simulink model "Simulations_Ex_2_3_4_5"  (R2016b)
settings: Solver=VariableStepAuto  StartTime=0.0  StopTime=25  RelTol=1e-3
libraries: powerlib_meascontrol x5
settings Model: Creator=CBalla  LastModifiedBy=CBalla

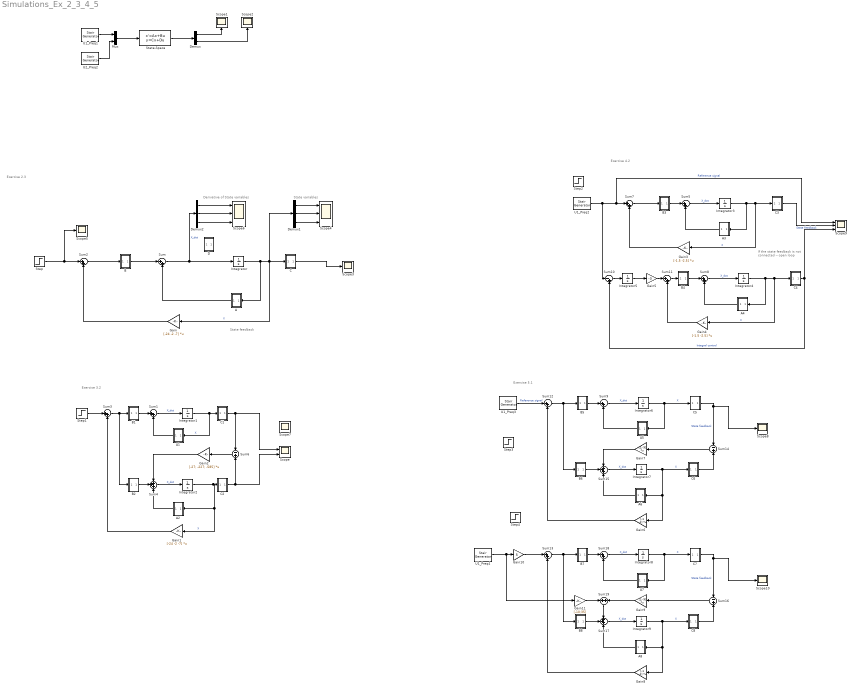
== system Simulations_Ex_2_3_4_5 ==
  note: If the state feedback is not
      | connected -- open loop
  note: Exercise 2.3
  note: State feedback
  note: Derivative of State variables
  note: State variables
  note: Exercise 3.2
  note: Exercise 4.2
  note: Exercise 5.1
  A : Subsystem
      mask Display:
      | %color('cyan')
      | color('magenta')
      | disp('{\bf\fontsize{14}A}', 'texmode','on');
      | %disp('B')
  A1 : Subsystem
      mask Display:
      | %color('cyan')
      | color('magenta')
      | disp('{\bf\fontsize{14}A}', 'texmode','on');
      | %disp('B')
  A2 : Subsystem
      mask Display:
      | %color('cyan')
      | color('magenta')
      | disp('{\bf\fontsize{14}A}', 'texmode','on');
      | %disp('B')
  A3 : Subsystem
      mask Display:
      | %color('cyan')
      | color('magenta')
      | disp('{\bf\fontsize{14}A}', 'texmode','on');
      | %disp('B')
  A4 : Subsystem
      mask Display:
      | %color('cyan')
      | color('magenta')
      | disp('{\bf\fontsize{14}A}', 'texmode','on');
      | %disp('B')
  A5 : Subsystem
      mask Display:
      | %color('cyan')
      | color('magenta')
      | disp('{\bf\fontsize{14}A}', 'texmode','on');
      | %disp('B')
  A6 : Subsystem
      mask Display:
      | %color('cyan')
      | color('magenta')
      | disp('{\bf\fontsize{14}A}', 'texmode','on');
      | %disp('B')
  A7 : Subsystem
      mask Display:
      | %color('cyan')
      | color('magenta')
      | disp('{\bf\fontsize{14}A}', 'texmode','on');
      | %disp('B')
  A8 : Subsystem
      mask Display:
      | %color('cyan')
      | color('magenta')
      | disp('{\bf\fontsize{14}A}', 'texmode','on');
      | %disp('B')
  B : Subsystem
      mask Display:
      | %color('cyan')
      | color('magenta')
      | disp('{\bf\fontsize{14}B}', 'texmode','on');
      | %disp('B')
  B1 : Subsystem
      mask Display:
      | %color('cyan')
      | color('magenta')
      | disp('{\bf\fontsize{14}B}', 'texmode','on');
      | %disp('B')
  B2 : Subsystem
      mask Display:
      | %color('cyan')
      | color('magenta')
      | disp('{\bf\fontsize{14}B}', 'texmode','on');
      | %disp('B')
  B3 : Subsystem
      mask Display:
      | %color('cyan')
      | color('magenta')
      | disp('{\bf\fontsize{14}B}', 'texmode','on');
      | %disp('B')
  B4 : Subsystem
      mask Display:
      | %color('cyan')
      | color('magenta')
      | disp('{\bf\fontsize{14}B}', 'texmode','on');
      | %disp('B')
  B5 : Subsystem
      mask Display:
      | %color('cyan')
      | color('magenta')
      | disp('{\bf\fontsize{14}B}', 'texmode','on');
      | %disp('B')
  B6 : Subsystem
      mask Display:
      | %color('cyan')
      | color('magenta')
      | disp('{\bf\fontsize{14}B}', 'texmode','on');
      | %disp('B')
  B7 : Subsystem
      mask Display:
      | %color('cyan')
      | color('magenta')
      | disp('{\bf\fontsize{14}B}', 'texmode','on');
      | %disp('B')
  B8 : Subsystem
      mask Display:
      | %color('cyan')
      | color('magenta')
      | disp('{\bf\fontsize{14}B}', 'texmode','on');
      | %disp('B')
  C : Subsystem
      mask Display:
      | %color('cyan')
      | color('magenta')
      | disp('{\bf\fontsize{14}C}', 'texmode','on');
      | %disp('B')
  C1 : Subsystem
      mask Display:
      | %color('cyan')
      | color('magenta')
      | disp('{\bf\fontsize{14}C}', 'texmode','on');
      | %disp('B')
  C2 : Subsystem
      mask Display:
      | %color('cyan')
      | color('magenta')
      | disp('{\bf\fontsize{14}C}', 'texmode','on');
      | %disp('B')
  C3 : Subsystem
      mask Display:
      | %color('cyan')
      | color('magenta')
      | disp('{\bf\fontsize{14}C}', 'texmode','on');
      | %disp('B')
  C4 : Subsystem
      mask Display:
      | %color('cyan')
      | color('magenta')
      | disp('{\bf\fontsize{14}C}', 'texmode','on');
      | %disp('B')
  C5 : Subsystem
      mask Display:
      | %color('cyan')
      | color('magenta')
      | disp('{\bf\fontsize{14}C}', 'texmode','on');
      | %disp('B')
  C6 : Subsystem
      mask Display:
      | %color('cyan')
      | color('magenta')
      | disp('{\bf\fontsize{14}C}', 'texmode','on');
      | %disp('B')
  C7 : Subsystem
      mask Display:
      | %color('cyan')
      | color('magenta')
      | disp('{\bf\fontsize{14}C}', 'texmode','on');
      | %disp('B')
  C8 : Subsystem
      mask Display:
      | %color('cyan')
      | color('magenta')
      | disp('{\bf\fontsize{14}C}', 'texmode','on');
      | %disp('B')
  D : Subsystem
      mask Display:
      | %color('cyan')
      | color('magenta')
      | disp('{\bf\fontsize{14}D}', 'texmode','on');
      | %disp('B')
  Demux : Demux  Outputs=2
  Demux1 : Demux  Outputs=3
  Demux2 : Demux  Outputs=3
  Gain : Gain  Gain=[-24 -2 -7]  Multiplication=Matrix(K*u)
  Gain1 : Gain  Gain=[-24 -2 -7]  Multiplication=Matrix(K*u)
  Gain10 : Gain  Gain=5
  Gain11 : Gain  Gain=[-10;35]
  Gain2 : Gain  Gain=[-27; -227; -585]  Multiplication=Matrix(K*u)
  Gain3 : Gain  Gain=[-1.5 -2.5]  Multiplication=Matrix(K*u)
  Gain4 : Gain  Gain=[-1.5 -2.5]  Multiplication=Matrix(K*u)
  Gain5 : Gain  Gain=-3
  Gain6 : Gain  Gain=[-1 -1]  Multiplication=Matrix(K*u)
  Gain7 : Gain  Gain=[2;-9]  Multiplication=Matrix(K*u)
  Gain8 : Gain  Gain=[-1 -1]  Multiplication=Matrix(K*u)
  Gain9 : Gain  Gain=[2;-9]  Multiplication=Matrix(K*u)
  Integrator{,2..9} (9 alike) : Integrator
  Integrator1 : Integrator  InitialCondition=-1
  Mux : Mux  Inputs=2
  Scope : Scope  NumInputPorts=2
  Scope{1..3,5,7..8,10} (7 alike) : Scope
  Scope4 : Scope  NumInputPorts=3
  Scope6 : Scope  NumInputPorts=3
  Scope9 : Scope  NumInputPorts=3
  State-Space : StateSpace  A=[-5.2159 -79.1175 -0.7209 -0.7209; 1 0 0 0; 0 0 -1.4430 -0.7209; 0 0 1 0]  B=|  C=|  D=[0.9645 0; 0 0]  X0=0
      B=|
      | [1 0;
      | 0 0;
      | 0 1; 0 0]
      C=|
      | [-1.3307 2.8087 -0.69530805 -0.69530805;
      | 0 0 0.7209 0.7209]
  Step{,1..4} (5 alike) : Step  Time=3  SampleTime=0
  Sum{,1..3,5,7..9,11..13,18} (12 alike) : Sum  Inputs=|++
  Sum10 : Sum  Inputs=|-+
  Sum14 : Sum  Inputs=-+
  Sum15 : Sum  Inputs=+++
  Sum16 : Sum  Inputs=-+
  Sum17 : Sum  Inputs=+++
  Sum19 : Sum
  Sum4 : Sum  Inputs=+++
  Sum6 : Sum  Inputs=-+
  U1_Preq1 : powerlib_meascontrol/Pulse & Signal Generators/Stair Generator  t=[4, 7, 12, 18,25]  e=[10000, 11500, 2000, 15000,2000]  Ts=0
  U1_Preq2 : powerlib_meascontrol/Pulse & Signal Generators/Stair Generator  t=[1, 4, 10, 15,20]  e=[1, 0, 2, -1,0]  Ts=0
  U1_Preq3 : powerlib_meascontrol/Pulse & Signal Generators/Stair Generator  t=[1, 4, 10, 15,20]  e=[1, 0, 2, -1,0]  Ts=0
  U1_Preq4 : powerlib_meascontrol/Pulse & Signal Generators/Stair Generator  t=[1, 4, 10, 15,20]  e=[1, 0, 2, -1,0]  Ts=0
  U2_Preq2 : powerlib_meascontrol/Pulse & Signal Generators/Stair Generator  t=[10, 18,25]  e=[10000, 15000,2000]  Ts=0
  wires:
  U1_Preq1/1 -> Mux/1
  U2_Preq2/1 -> Mux/2
  Mux/1 -> State-Space/1
  State-Space/1 -> Demux/1
  Demux/1 -> Scope1/1
  Demux/2 -> Scope2/1
  B/1(Out1) -> Sum/1
  A/1(Out1) -> Sum/2
  Demux2/1 -> Scope6/1
  Demux2/2 -> Scope6/2
  Demux2/3 -> Scope6/3
  Sum2/1 -> B/1(In1)
  Integrator/1 -> Demux1/1, Gain/1, C/1(In1), A/1(In1)  "X"
  Gain/1 -> Sum2/2
  Sum/1 -> Demux2/1, Integrator/1  "X_dot"
  C/1(Out1) -> Scope3/1
  Step/1 -> Scope5/1, Sum2/1
  Demux1/2 -> Scope4/2
  Demux1/3 -> Scope4/3
  Demux1/1 -> Scope4/1
  B1/1(Out1) -> Sum1/1
  A1/1(Out1) -> Sum1/2
  Sum3/1 -> B2/1(In1), B1/1(In1)
  Integrator1/1 -> C1/1(In1), A1/1(In1)  "X"
  Sum1/1 -> Integrator1/1  "X_dot"
  C1/1(Out1) -> Sum6/1, Scope/1
  Step1/1 -> Sum3/1
  Integrator2/1 -> Gain1/1, A2/1(In1), C2/1(In1)  "X"
  Sum4/1 -> Integrator2/1  "X_dot"
  C2/1(Out1) -> Scope/2, Sum6/2
  Gain1/1 -> Sum3/2
  Sum6/1 -> Gain2/1
  A2/1(Out1) -> Sum4/3
  B2/1(Out1) -> Sum4/2
  Gain2/1 -> Sum4/1
  B3/1(Out1) -> Sum5/1
  A3/1(Out1) -> Sum5/2
  Sum7/1 -> B3/1(In1)
  Integrator3/1 -> Gain3/1, C3/1(In1), A3/1(In1)  "X"
  Sum5/1 -> Integrator3/1  "X_dot"
  U1_Preq2/1 -> Sum10/1, Scope9/1, Sum7/1  "Reference signal"
  C3/1(Out1) -> Scope9/2  "State feedback"
  B4/1(Out1) -> Sum8/1
  A4/1(Out1) -> Sum8/2
  Sum10/1 -> Integrator5/1
  Integrator4/1 -> Gain4/1, C4/1(In1), A4/1(In1)  "X"
  Sum8/1 -> Integrator4/1  "X_dot"
  Integrator5/1 -> Gain5/1
  Gain5/1 -> Sum11/1
  Sum11/1 -> B4/1(In1)
  Gain4/1 -> Sum11/2
  C4/1(Out1) -> Scope9/3, Sum10/2  "Integral control"
  Gain3/1 -> Sum7/2
  B5/1(Out1) -> Sum9/1
  A5/1(Out1) -> Sum9/2
  Integrator6/1 -> C5/1(In1), A5/1(In1)  "X"
  Sum9/1 -> Integrator6/1  "X_dot"
  B6/1(Out1) -> Sum15/2
  Sum12/1 -> B6/1(In1), B5/1(In1)
  Integrator7/1 -> C6/1(In1), Gain6/1, A6/1(In1)  "X"
  Sum15/1 -> Integrator7/1  "X_dot"
  C5/1(Out1) -> Scope8/1, Sum14/1  "State feedback"
  C6/1(Out1) -> Sum14/2
  Sum14/1 -> Gain7/1
  A6/1(Out1) -> Sum15/3
  Gain7/1 -> Sum15/1
  Gain6/1 -> Sum12/2
  B7/1(Out1) -> Sum18/1
  A7/1(Out1) -> Sum18/2
  Integrator8/1 -> C7/1(In1), A7/1(In1)  "X"
  Sum18/1 -> Integrator8/1  "X_dot"
  B8/1(Out1) -> Sum17/2
  Sum13/1 -> B8/1(In1), B7/1(In1)
  Integrator9/1 -> C8/1(In1), Gain8/1, A8/1(In1)  "X"
  Sum17/1 -> Integrator9/1  "X_dot"
  C7/1(Out1) -> Scope10/1, Sum16/1  "State feedback"
  C8/1(Out1) -> Sum16/2
  Sum16/1 -> Gain9/1
  A8/1(Out1) -> Sum17/3
  Gain8/1 -> Sum13/2
  U1_Preq3/1 -> Sum12/1  "Reference signal"
  U1_Preq4/1 -> Gain11/1, Gain10/1
  Gain10/1 -> Sum13/1
  Sum19/1 -> Sum17/1
  Gain9/1 -> Sum19/2
  Gain11/1 -> Sum19/1

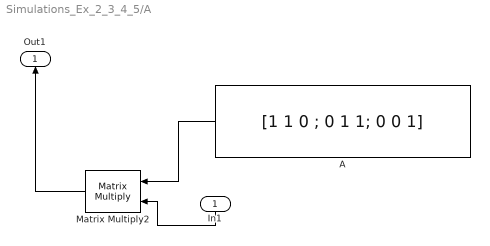
== system Simulations_Ex_2_3_4_5/A ==
  In1 : Inport
  A : Constant  Value=[1 1 0 ; 0 1 1; 0 0 1]  VectorParams1D=off
  Matrix Multiply2 : Product  Multiplication=Matrix(*)
  Out1 : Outport
  wires:
  Matrix Multiply2/1 -> Out1/1
  A/1 -> Matrix Multiply2/1
  In1/1 -> Matrix Multiply2/2

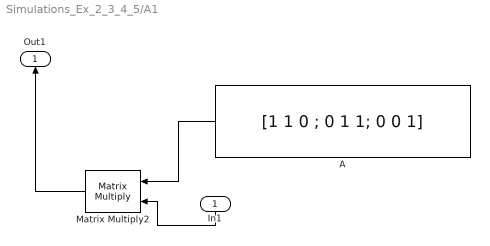
== system Simulations_Ex_2_3_4_5/A1 ==
  In1 : Inport
  A : Constant  Value=[1 1 0 ; 0 1 1; 0 0 1]  VectorParams1D=off
  Matrix Multiply2 : Product  Multiplication=Matrix(*)
  Out1 : Outport
  wires:
  Matrix Multiply2/1 -> Out1/1
  A/1 -> Matrix Multiply2/1
  In1/1 -> Matrix Multiply2/2

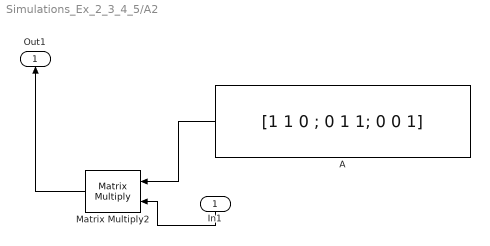
== system Simulations_Ex_2_3_4_5/A2 ==
  In1 : Inport
  A : Constant  Value=[1 1 0 ; 0 1 1; 0 0 1]  VectorParams1D=off
  Matrix Multiply2 : Product  Multiplication=Matrix(*)
  Out1 : Outport
  wires:
  Matrix Multiply2/1 -> Out1/1
  A/1 -> Matrix Multiply2/1
  In1/1 -> Matrix Multiply2/2

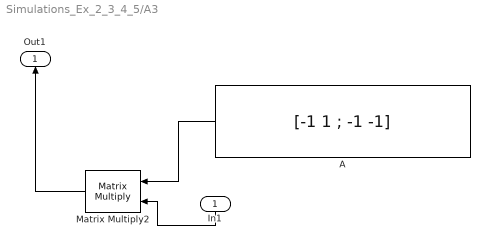
== system Simulations_Ex_2_3_4_5/A3 ==
  In1 : Inport
  A : Constant  Value=[-1 1 ; -1 -1]  VectorParams1D=off
  Matrix Multiply2 : Product  Multiplication=Matrix(*)
  Out1 : Outport
  wires:
  Matrix Multiply2/1 -> Out1/1
  A/1 -> Matrix Multiply2/1
  In1/1 -> Matrix Multiply2/2

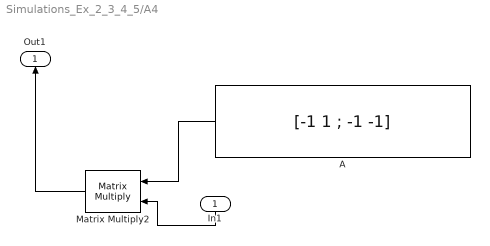
== system Simulations_Ex_2_3_4_5/A4 ==
  In1 : Inport
  A : Constant  Value=[-1 1 ; -1 -1]  VectorParams1D=off
  Matrix Multiply2 : Product  Multiplication=Matrix(*)
  Out1 : Outport
  wires:
  Matrix Multiply2/1 -> Out1/1
  A/1 -> Matrix Multiply2/1
  In1/1 -> Matrix Multiply2/2

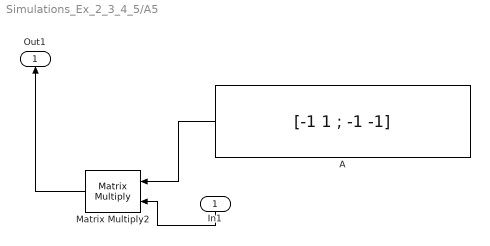
== system Simulations_Ex_2_3_4_5/A5 ==
  In1 : Inport
  A : Constant  Value=[-1 1 ; -1 -1]  VectorParams1D=off
  Matrix Multiply2 : Product  Multiplication=Matrix(*)
  Out1 : Outport
  wires:
  Matrix Multiply2/1 -> Out1/1
  A/1 -> Matrix Multiply2/1
  In1/1 -> Matrix Multiply2/2

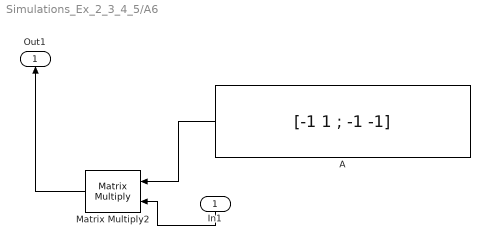
== system Simulations_Ex_2_3_4_5/A6 ==
  In1 : Inport
  A : Constant  Value=[-1 1 ; -1 -1]  VectorParams1D=off
  Matrix Multiply2 : Product  Multiplication=Matrix(*)
  Out1 : Outport
  wires:
  Matrix Multiply2/1 -> Out1/1
  A/1 -> Matrix Multiply2/1
  In1/1 -> Matrix Multiply2/2

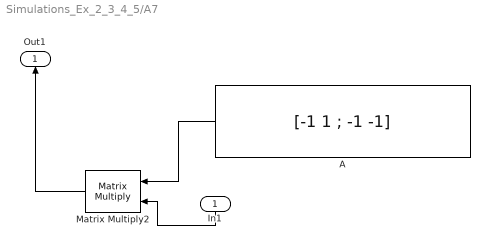
== system Simulations_Ex_2_3_4_5/A7 ==
  In1 : Inport
  A : Constant  Value=[-1 1 ; -1 -1]  VectorParams1D=off
  Matrix Multiply2 : Product  Multiplication=Matrix(*)
  Out1 : Outport
  wires:
  Matrix Multiply2/1 -> Out1/1
  A/1 -> Matrix Multiply2/1
  In1/1 -> Matrix Multiply2/2

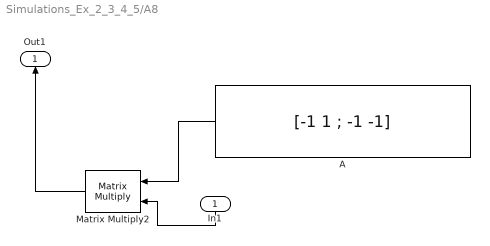
== system Simulations_Ex_2_3_4_5/A8 ==
  In1 : Inport
  A : Constant  Value=[-1 1 ; -1 -1]  VectorParams1D=off
  Matrix Multiply2 : Product  Multiplication=Matrix(*)
  Out1 : Outport
  wires:
  Matrix Multiply2/1 -> Out1/1
  A/1 -> Matrix Multiply2/1
  In1/1 -> Matrix Multiply2/2

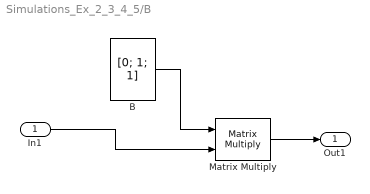
== system Simulations_Ex_2_3_4_5/B ==
  In1 : Inport
  B : Constant  Value=|  VectorParams1D=off
      | [0;
      | 1;
      | 1]
  Matrix Multiply : Product  Multiplication=Matrix(*)
  Out1 : Outport
  wires:
  Matrix Multiply/1 -> Out1/1
  B/1 -> Matrix Multiply/1
  In1/1 -> Matrix Multiply/2

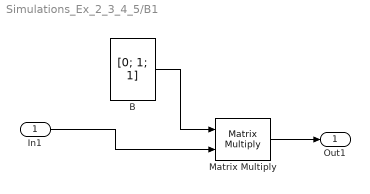
== system Simulations_Ex_2_3_4_5/B1 ==
  In1 : Inport
  B : Constant  Value=|  VectorParams1D=off
      | [0;
      | 1;
      | 1]
  Matrix Multiply : Product  Multiplication=Matrix(*)
  Out1 : Outport
  wires:
  Matrix Multiply/1 -> Out1/1
  B/1 -> Matrix Multiply/1
  In1/1 -> Matrix Multiply/2

== system Simulations_Ex_2_3_4_5/B2 ==
  In1 : Inport
  B : Constant  Value=|  VectorParams1D=off
      | [0;
      | 1;
      | 1]
  Matrix Multiply : Product  Multiplication=Matrix(*)
  Out1 : Outport
  wires:
  Matrix Multiply/1 -> Out1/1
  B/1 -> Matrix Multiply/1
  In1/1 -> Matrix Multiply/2

== system Simulations_Ex_2_3_4_5/B3 ==
  In1 : Inport
  B : Constant  Value=|  VectorParams1D=off
      | [1;
      | 1]
  Matrix Multiply : Product  Multiplication=Matrix(*)
  Out1 : Outport
  wires:
  Matrix Multiply/1 -> Out1/1
  B/1 -> Matrix Multiply/1
  In1/1 -> Matrix Multiply/2

== system Simulations_Ex_2_3_4_5/B4 ==
  In1 : Inport
  B : Constant  Value=|  VectorParams1D=off
      | [1;
      | 1]
  Matrix Multiply : Product  Multiplication=Matrix(*)
  Out1 : Outport
  wires:
  Matrix Multiply/1 -> Out1/1
  B/1 -> Matrix Multiply/1
  In1/1 -> Matrix Multiply/2

== system Simulations_Ex_2_3_4_5/B5 ==
  In1 : Inport
  B : Constant  Value=|  VectorParams1D=off
      | [1;
      | 1]
  Matrix Multiply : Product  Multiplication=Matrix(*)
  Out1 : Outport
  wires:
  Matrix Multiply/1 -> Out1/1
  B/1 -> Matrix Multiply/1
  In1/1 -> Matrix Multiply/2

== system Simulations_Ex_2_3_4_5/B6 ==
  In1 : Inport
  B : Constant  Value=|  VectorParams1D=off
      | [1;
      | 1]
  Matrix Multiply : Product  Multiplication=Matrix(*)
  Out1 : Outport
  wires:
  Matrix Multiply/1 -> Out1/1
  B/1 -> Matrix Multiply/1
  In1/1 -> Matrix Multiply/2

== system Simulations_Ex_2_3_4_5/B7 ==
  In1 : Inport
  B : Constant  Value=|  VectorParams1D=off
      | [1;
      | 1]
  Matrix Multiply : Product  Multiplication=Matrix(*)
  Out1 : Outport
  wires:
  Matrix Multiply/1 -> Out1/1
  B/1 -> Matrix Multiply/1
  In1/1 -> Matrix Multiply/2

== system Simulations_Ex_2_3_4_5/B8 ==
  In1 : Inport
  B : Constant  Value=|  VectorParams1D=off
      | [1;
      | 1]
  Matrix Multiply : Product  Multiplication=Matrix(*)
  Out1 : Outport
  wires:
  Matrix Multiply/1 -> Out1/1
  B/1 -> Matrix Multiply/1
  In1/1 -> Matrix Multiply/2

== system Simulations_Ex_2_3_4_5/C ==
  In1 : Inport
  C : Constant  Value=[1 0 0]  VectorParams1D=off
  Matrix Multiply1 : Product  Multiplication=Matrix(*)
  Out1 : Outport
  wires:
  Matrix Multiply1/1 -> Out1/1
  In1/1 -> Matrix Multiply1/2
  C/1 -> Matrix Multiply1/1

== system Simulations_Ex_2_3_4_5/C1 ==
  In1 : Inport
  C : Constant  Value=[1 0 0]  VectorParams1D=off
  Matrix Multiply1 : Product  Multiplication=Matrix(*)
  Out1 : Outport
  wires:
  Matrix Multiply1/1 -> Out1/1
  In1/1 -> Matrix Multiply1/2
  C/1 -> Matrix Multiply1/1

== system Simulations_Ex_2_3_4_5/C2 ==
  In1 : Inport
  C : Constant  Value=[1 0 0]  VectorParams1D=off
  Matrix Multiply1 : Product  Multiplication=Matrix(*)
  Out1 : Outport
  wires:
  Matrix Multiply1/1 -> Out1/1
  In1/1 -> Matrix Multiply1/2
  C/1 -> Matrix Multiply1/1

== system Simulations_Ex_2_3_4_5/C3 ==
  In1 : Inport
  C : Constant  Value=[1 0]  VectorParams1D=off
  Matrix Multiply1 : Product  Multiplication=Matrix(*)
  Out1 : Outport
  wires:
  Matrix Multiply1/1 -> Out1/1
  In1/1 -> Matrix Multiply1/2
  C/1 -> Matrix Multiply1/1

== system Simulations_Ex_2_3_4_5/C4 ==
  In1 : Inport
  C : Constant  Value=[1 0]  VectorParams1D=off
  Matrix Multiply1 : Product  Multiplication=Matrix(*)
  Out1 : Outport
  wires:
  Matrix Multiply1/1 -> Out1/1
  In1/1 -> Matrix Multiply1/2
  C/1 -> Matrix Multiply1/1

== system Simulations_Ex_2_3_4_5/C5 ==
  In1 : Inport
  C : Constant  Value=[1 1]  VectorParams1D=off
  Matrix Multiply1 : Product  Multiplication=Matrix(*)
  Out1 : Outport
  wires:
  Matrix Multiply1/1 -> Out1/1
  In1/1 -> Matrix Multiply1/2
  C/1 -> Matrix Multiply1/1

== system Simulations_Ex_2_3_4_5/C6 ==
  In1 : Inport
  C : Constant  Value=[1 1]  VectorParams1D=off
  Matrix Multiply1 : Product  Multiplication=Matrix(*)
  Out1 : Outport
  wires:
  Matrix Multiply1/1 -> Out1/1
  In1/1 -> Matrix Multiply1/2
  C/1 -> Matrix Multiply1/1

== system Simulations_Ex_2_3_4_5/C7 ==
  In1 : Inport
  C : Constant  Value=[1 1]  VectorParams1D=off
  Matrix Multiply1 : Product  Multiplication=Matrix(*)
  Out1 : Outport
  wires:
  Matrix Multiply1/1 -> Out1/1
  In1/1 -> Matrix Multiply1/2
  C/1 -> Matrix Multiply1/1

== system Simulations_Ex_2_3_4_5/C8 ==
  In1 : Inport
  C : Constant  Value=[1 1]  VectorParams1D=off
  Matrix Multiply1 : Product  Multiplication=Matrix(*)
  Out1 : Outport
  wires:
  Matrix Multiply1/1 -> Out1/1
  In1/1 -> Matrix Multiply1/2
  C/1 -> Matrix Multiply1/1

== system Simulations_Ex_2_3_4_5/D ==
  In1 : Inport
  D : Constant  Value=[0]  VectorParams1D=off
  Matrix Multiply3 : Product  Multiplication=Matrix(*)
  Out1 : Outport
  wires:
  D/1 -> Matrix Multiply3/1
  Matrix Multiply3/1 -> Out1/1
  In1/1 -> Matrix Multiply3/2
